simulink model "w2025b"  (R2025b)
settings: Solver=VariableStepAuto  StopTime=60
values from neighbouring files (symbols this model uses):
  b1 = 0.008    [definicje.m]
  J = 0.03    [definicje.m]
  kf = 1.8/6.5    (= 0.276923076923)    [definicje.m]
  Ra = 3.0724    [definicje.m]
  tau = La/Ra    (= 0.0214334071084)    [definicje.m]
  Tl = 1    [definicje.m]
  Ua = 100    [definicje.m]
settings Model: Creator=Student  LastModifiedBy=piotr
settings ModelReferenceCC: EnableRefExpFcnMdlSchedulingChecks=on
settings RTWCC: GPUComputeCapability=3.5
settings SimscapeCC: SimscapeLogDecimation=1  SimscapeLogDataHistory=5000

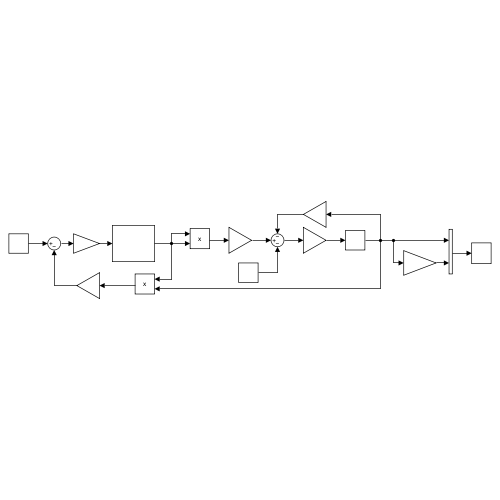
[thumbnail: Simulink's stored preview of the top-level diagram]
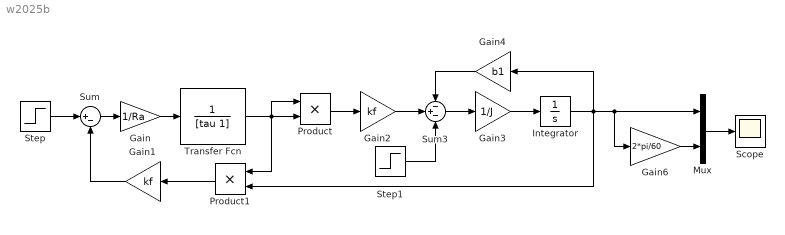
== system w2025b ==
  Gain : Gain  Gain=1/Ra
  Gain1 : Gain  Gain=kf
  Gain2 : Gain  Gain=kf
  Gain3 : Gain  Gain=1/J
  Gain4 : Gain  Gain=b1
  Gain6 : Gain  Gain=2*pi/60
  Integrator : Integrator
  Mux : Mux  Inputs=2
  Product : Product
  Product1 : Product
  Scope : Scope
      settings: ActiveDisplayYMinimum=-4.4061958405151529  ActiveDisplayYMaximum=260.467987303473
  Step : Step  After=Ua  SampleTime=0
  Step1 : Step  After=Tl  SampleTime=0
  Sum : Sum  Inputs=|+-
  Sum3 : Sum  Inputs=-+-
  Transfer Fcn : TransferFcn  Denominator=[tau 1]
  wires:
  Sum/1 -> Gain/1
  Gain/1 -> Transfer Fcn/1
  Gain2/1 -> Sum3/2
  Sum3/1 -> Gain3/1
  Gain3/1 -> Integrator/1
  Integrator/1 -> Gain6/1, Mux/1, Gain4/1, Product1/2
  Gain4/1 -> Sum3/1
  Gain6/1 -> Mux/2
  Mux/1 -> Scope/1
  Step/1 -> Sum/1
  Product/1 -> Gain2/1
  Transfer Fcn/1 -> Product/2, Product1/1, Product/1
  Product1/1 -> Gain1/1
  Gain1/1 -> Sum/2
  Step1/1 -> Sum3/3
